simulink library "ClairvauxLibrary"  (R2020b)
settings: Solver=VariableStepAuto  StartTime=0.0  StopTime=10.0  RelTol=1e-3
undefined symbols (not defined in the file): OutMax, OutMin, Ts, w0
libraries: $bdroot x4, simulink x2, sharedtransform x2
(part 2 of 2)

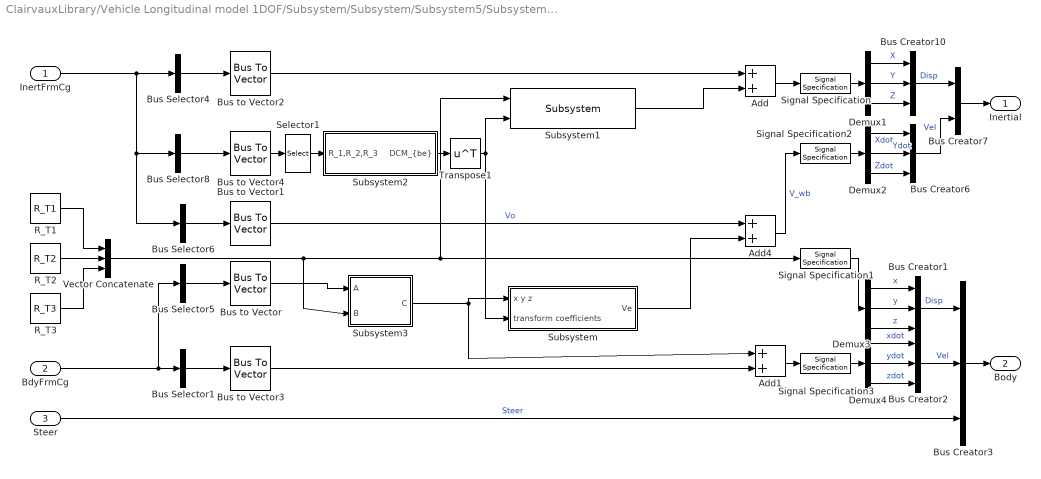
== system ClairvauxLibrary/Vehicle Longitudinal model 1DOF/Subsystem/Subsystem/Subsystem5/Subsystem/Subsystem ==
  InertFrmCg : Inport
  BdyFrmCg : Inport  Port=2
  Steer : Inport  Port=3
  Add : Sum
  Add1 : Sum
  Add4 : Sum
  Bus Creator{1..3,6,10} (5 alike) : BusCreator  Inputs=3
  Bus Creator7 : BusCreator  Inputs=2
  Bus Selector1 : BusSelector  OutputSignals=Vel.xdot,Vel.ydot,Vel.zdot  OutputAsBus=on
  Bus Selector4 : BusSelector  OutputSignals=Disp.X,Disp.Y,Disp.Z  OutputAsBus=on
  Bus Selector5 : BusSelector  OutputSignals=AngVel.p,AngVel.q,AngVel.r  OutputAsBus=on
  Bus Selector6 : BusSelector  OutputSignals=Vel.Xdot,Vel.Ydot,Vel.Zdot  OutputAsBus=on
  Bus Selector8 : BusSelector  OutputSignals=Ang.phi,Ang.theta,Ang.psi  OutputAsBus=on
  Bus to Vector{,1..4} (5 alike) : BusToVector
  Demux{1..4} (4 alike) : Demux  Outputs=3
  R_T1 : Constant  Value=R_T1
  R_T2 : Constant  Value=R_T2
  R_T3 : Constant  Value=R_T3
  Selector1 : Selector  InputPortWidth=3  IndexOptions=Index vector (dialog)  Indices=[3 2 1]  OutputSizes=1
  Signal Specification : SignalSpecification  Unit=m
  Signal Specification1 : SignalSpecification  Unit=m
  Signal Specification2 : SignalSpecification  Unit=m/s
  Signal Specification3 : SignalSpecification  Unit=m/s
  Subsystem : Subsystem
  Subsystem1 : $bdroot/Vehicle Longitudinal model 1DOF/Subsystem/Subsystem/Subsystem5/Subsystem/Subsystem/Subsystem  SystemSampleTime=-1  VariantActivationTime=update diagram  Latency=0  AutoFrameSizeCalculation=off
  Subsystem2 : Subsystem
  Subsystem3 : Subsystem
  Transpose1 : Math  Operator=transpose  SignedPower=on  SaturateOnIntegerOverflow=on
  Vector Concatenate : Concatenate  NumInputs=3
  Inertial : Outport  VectorParamsAs1DForOutWhenUnconnected=off
  Body : Outport  Port=2  VectorParamsAs1DForOutWhenUnconnected=off
  wires:
  Demux1/1 -> Bus Creator10/1  "X"
  Bus Selector8/1 -> Bus to Vector4/1
  Subsystem2/1("DCM_{be}") -> Transpose1/1
  Steer/1 -> Bus Creator3/3  "Steer"
  R_T3/1 -> Vector Concatenate/3
  Subsystem1/1 -> Add/2
  Demux2/3 -> Bus Creator6/3  "Zdot"
  Signal Specification3/1 -> Demux4/1
  Add/1 -> Signal Specification/1
  Demux3/2 -> Bus Creator1/2  "y"
  Selector1/1 -> Subsystem2/1(R_1,R_2,R_3)
  Signal Specification1/1 -> Demux3/1
  InertFrmCg/1 -> Bus Selector8/1, Bus Selector6/1, Bus Selector4/1
  Bus to Vector1/1 -> Add4/1  "Vo"
  Bus Selector5/1 -> Bus to Vector/1
  Bus to Vector/1 -> Subsystem3/1(A)
  Bus to Vector2/1 -> Add/1
  Add4/1 -> Signal Specification2/1  "V_wb"
  Bus Selector6/1 -> Bus to Vector1/1
  BdyFrmCg/1 -> Bus Selector1/1, Bus Selector5/1
  Bus to Vector3/1 -> Add1/2
  Subsystem3/1(C) -> Add1/1, Subsystem/1(x y z)
  Bus Creator7/1 -> Inertial/1
  Bus Selector4/1 -> Bus to Vector2/1
  Demux3/1 -> Bus Creator1/1  "x"
  Bus Creator1/1 -> Bus Creator3/1  "Disp"
  Bus Creator2/1 -> Bus Creator3/2  "Vel"
  Demux4/2 -> Bus Creator2/2  "ydot"
  Demux2/1 -> Bus Creator6/1  "Xdot"
  Demux4/3 -> Bus Creator2/3  "zdot"
  Demux1/2 -> Bus Creator10/2  "Y"
  Demux2/2 -> Bus Creator6/2  "Ydot"
  Signal Specification2/1 -> Demux2/1
  Bus Creator6/1 -> Bus Creator7/2  "Vel"
  Bus Creator10/1 -> Bus Creator7/1  "Disp"
  Bus Creator3/1 -> Body/1
  Signal Specification/1 -> Demux1/1
  Bus Selector1/1 -> Bus to Vector3/1
  Add1/1 -> Signal Specification3/1
  R_T2/1 -> Vector Concatenate/2
  Transpose1/1 -> Subsystem1/2, Subsystem/2(transform coefficients)
  Vector Concatenate/1 -> Subsystem3/2(B), Subsystem1/1, Signal Specification1/1
  Subsystem/1(Ve) -> Add4/2
  Demux4/1 -> Bus Creator2/1  "xdot"
  R_T1/1 -> Vector Concatenate/1
  Demux3/3 -> Bus Creator1/3  "z"
  Bus to Vector4/1 -> Selector1/1
  Demux1/3 -> Bus Creator10/3  "Z"

== system ClairvauxLibrary/Vehicle Longitudinal model 1DOF/Subsystem/Subsystem/Subsystem5/Subsystem/Subsystem/Subsystem ==
  x y z : Inport
  transform coefficients : Inport  Port=2
  Product : Product  Multiplication=Matrix(*)  InputSameDT=on  SaturateOnIntegerOverflow=on  OutDataTypeStr=Inherit: Same as first input
  Reshape1 : Reshape  OutputDimensionality=Column vector (2-D)
  Reshape2 : Reshape
  Ve : Outport  VectorParamsAs1DForOutWhenUnconnected=off
  wires:
  Reshape1/1 -> Product/2
  transform coefficients/1 -> Product/1
  x y z/1 -> Reshape1/1
  Product/1 -> Reshape2/1
  Reshape2/1 -> Ve/1

== system ClairvauxLibrary/Vehicle Longitudinal model 1DOF/Subsystem/Subsystem/Subsystem5/Subsystem/Subsystem/Subsystem2 ==
  R_1,R_2,R_3 : Inport  Unit=rad  PortDimensions=3
  Fcn11 : Fcn  Expr=u(5)*u(4)
  Fcn12 : Fcn  Expr=u(5)*u(1)
  Fcn13 : Fcn  Expr=-u(2)
  Fcn21 : Fcn  Expr=u(3)*u(2)*u(4) - u(6)*u(1)
  Fcn22 : Fcn  Expr=u(3)*u(2)*u(1) + u(6)*u(4)
  Fcn23 : Fcn  Expr=u(3)*u(5)
  Fcn31 : Fcn  Expr=u(6)*u(2)*u(4) + u(3)*u(1)
  Fcn32 : Fcn  Expr=u(6)*u(2)*u(1) - u(3)*u(4)
  Fcn33 : Fcn  Expr=u(6)*u(5)
  Mux : Mux  Inputs=2
  Subsystem : Subsystem
  sincos : Trigonometry  Operator=sincos
  "DCM_{be}" : Outport  Unit=1  PortDimensions=[3,3]  VectorParamsAs1DForOutWhenUnconnected=off
  wires:
  Fcn22/1 -> Subsystem/5(M22)
  Fcn21/1 -> Subsystem/4(M21)
  Fcn31/1 -> Subsystem/7(M31)
  Mux/1 -> Fcn11/1, Fcn12/1, Fcn13/1, Fcn21/1, Fcn32/1, Fcn33/1, Fcn31/1, Fcn23/1, Fcn22/1
  Fcn23/1 -> Subsystem/6(M23)
  Fcn33/1 -> Subsystem/9(M33)
  Fcn32/1 -> Subsystem/8(M32)
  Fcn12/1 -> Subsystem/2(M12)
  Subsystem/1(Matrix) -> "DCM_{be}"/1
  sincos/1 -> Mux/1
  Fcn11/1 -> Subsystem/1(M11)
  Fcn13/1 -> Subsystem/3(M13)
  sincos/2 -> Mux/2
  R_1,R_2,R_3/1 -> sincos/1

== system ClairvauxLibrary/Vehicle Longitudinal model 1DOF/Subsystem/Subsystem/Subsystem5/Subsystem/Subsystem/Subsystem3 ==
  A : Inport
  B : Inport  Port=2
  "A " : InportShadow
  "B " : InportShadow  Port=2
  Subsystem1 : $bdroot/Vehicle Longitudinal model 1DOF/Subsystem/Subsystem/Subsystem5/Subsystem/Subsystem/Subsystem3/Subsystem2  SystemSampleTime=-1  VariantActivationTime=update diagram  Latency=0  AutoFrameSizeCalculation=off
  Subsystem2 : Subsystem
  Sum : Sum  Inputs=+|-  InputSameDT=on  SaturateOnIntegerOverflow=on  OutDataTypeStr=Inherit: Same as first input
  C : Outport  VectorParamsAs1DForOutWhenUnconnected=off
  wires:
  B/1 -> Subsystem2/2(B)
  Sum/1 -> C/1
  Subsystem1/1 -> Sum/2
  A/1 -> Subsystem2/1(A)
  "A "/1 -> Subsystem1/1
  "B "/1 -> Subsystem1/2
  Subsystem2/1(Out1) -> Sum/1

== system ClairvauxLibrary/Vehicle Longitudinal model 1DOF/Subsystem/Subsystem/Subsystem5/Subsystem/Subsystem/Subsystem2/Subsystem ==
  M11 : Inport  PortDimensions=1
  M12 : Inport  Port=2  PortDimensions=1
  M13 : Inport  Port=3  PortDimensions=1
  M21 : Inport  Port=4  PortDimensions=1
  M22 : Inport  Port=5  PortDimensions=1
  M23 : Inport  Port=6  PortDimensions=1
  M31 : Inport  Port=7  PortDimensions=1
  M32 : Inport  Port=8  PortDimensions=1
  M33 : Inport  Port=9  PortDimensions=1
  Reshape (9) to [3x3] column-major : Reshape  OutputDimensionality=Customize  OutputDimensions=[3,3]
  Vector Concatenate : Concatenate  NumInputs=9
  Matrix : Outport  PortDimensions=[3 3]  VectorParamsAs1DForOutWhenUnconnected=off
  wires:
  M11/1 -> Vector Concatenate/1
  M12/1 -> Vector Concatenate/4
  M32/1 -> Vector Concatenate/6
  M13/1 -> Vector Concatenate/7
  Reshape (9) to [3x3] column-major/1 -> Matrix/1
  Vector Concatenate/1 -> Reshape (9) to [3x3] column-major/1
  M22/1 -> Vector Concatenate/5
  M23/1 -> Vector Concatenate/8
  M31/1 -> Vector Concatenate/3
  M21/1 -> Vector Concatenate/2
  M33/1 -> Vector Concatenate/9

== system ClairvauxLibrary/Vehicle Longitudinal model 1DOF/Subsystem/Subsystem/Subsystem5/Subsystem/Subsystem/Subsystem3/Subsystem2 ==
  A : Inport
  B : Inport  Port=2
  Demux : Demux  Outputs=3
  Demux1 : Demux  Outputs=3
  Mux : Mux  Inputs=3
  i x j : Product  InputSameDT=on  SaturateOnIntegerOverflow=on  OutDataTypeStr=Inherit: Same as first input
  j x k : Product  InputSameDT=on  SaturateOnIntegerOverflow=on  OutDataTypeStr=Inherit: Same as first input
  k x i : Product  InputSameDT=on  SaturateOnIntegerOverflow=on  OutDataTypeStr=Inherit: Same as first input
  Out1 : Outport  VectorParamsAs1DForOutWhenUnconnected=off
  wires:
  B/1 -> Demux1/1
  i x j/1 -> Mux/3
  Demux/2 -> j x k/1
  Mux/1 -> Out1/1
  Demux1/1 -> k x i/2
  j x k/1 -> Mux/1
  Demux/1 -> i x j/1
  Demux/3 -> k x i/1
  Demux1/2 -> i x j/2
  A/1 -> Demux/1
  k x i/1 -> Mux/2
  Demux1/3 -> j x k/2

== matlab function ClairvauxLibrary/DiscreteSecondOrderSection/MATLAB Function ==
  data: w input; a output; zeta input; tau input; b output; c output
function [a,b,c] = fcn(w,zeta,tau)
% Formulas for Tustin discretization of w^2/(s^2 + 2*zeta*w*s + s^2)
%#codegen
wt = tau*w;    % w*tau
p = 2*zeta*wt;
q = wt^2;
r = 1+q;
d = p+r;
a = q/d;       % wt^2/(1+2*zeta*wt+wt^2)
b = (1-q)/d;   % (1-wt^2)/(1+2*zeta*wt+wt^2)
c = (r-p)/d;   % (1-2*zeta*wt+wt^2)/(1+2*zeta*wt+wt^2)
